simulink model "untitled"  (R2018b)
settings: Solver=VariableStepAuto  StartTime=0.0  StopTime=10.0  RelTol=1e-3
libraries: vrlib x2
settings Model: Creator=Notebook  LastModifiedBy=Notebook

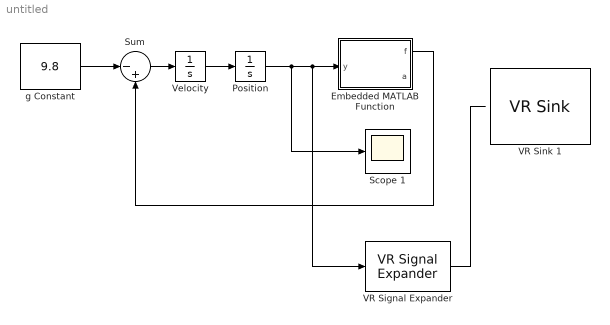
== system untitled ==
  Embedded MATLAB Function : MATLAB Function  TreatAsAtomicUnit=on
  Position : Integrator
  Scope 1 : Scope
  Sum : Sum  Inputs=|-+
  VR Signal Expander : vrlib/VR Signal Expander  outwidth=4  outidx=[2 4]
      settings: SourceProductName=Simulink 3D Animation  SourceProductBaseCode=VR
  VR Sink 1 : vrlib/VR Sink  InstantiateOnLoad=on  SampleTime=0.1  ViewEnable=on  RemoteChange=off  RemoteView=on  AutoView=off  VideoDimensions=[]  AllowVariableSize=off
      settings: SourceProductBaseCode=VR
  Velocity : Integrator
  g Constant : Constant  Value=9.8
  wires:
  g Constant/1 -> Sum/1
  Sum/1 -> Velocity/1
  Velocity/1 -> Position/1
  Embedded MATLAB Function/1(f) -> Sum/2
  Position/1 -> VR Signal Expander/1, Embedded MATLAB Function/1(y), Scope 1/1
  VR Signal Expander/1 -> ?

== matlab function untitled/Embedded MATLAB Function ==
  data: y input; f output; a output
function [f, a]= fcn(y)
if y<1e-4
    y=1e-4;
end
if y<1.5
    f=500*(1.5-y)
    a=sqrt(1.5^3/y);
else
    f=0;
    a=1.5;
end
